simulink model "Deadbeat_controller"  (R2021b)
settings: Solver=ode45  StartTime=0.0  StopTime=0.5  RelTol=1e-3
values from neighbouring files (symbols this model uses):
  G1 = 1/(R + L*s)    [Project.m]
  G2 = Kt/(m*s^2 + c*s + k)    [Project.m]
  Gd_db = minreal(Fz/(Gz * (1 - Fz)))    [Project.m]
  Ts = 0.02    [Project.m]
settings Model: Creator=Amir  LastModifiedBy=Amir

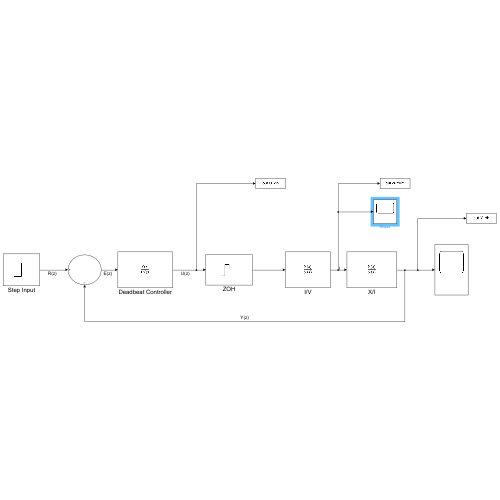
[thumbnail: Simulink's stored preview of the top-level diagram]
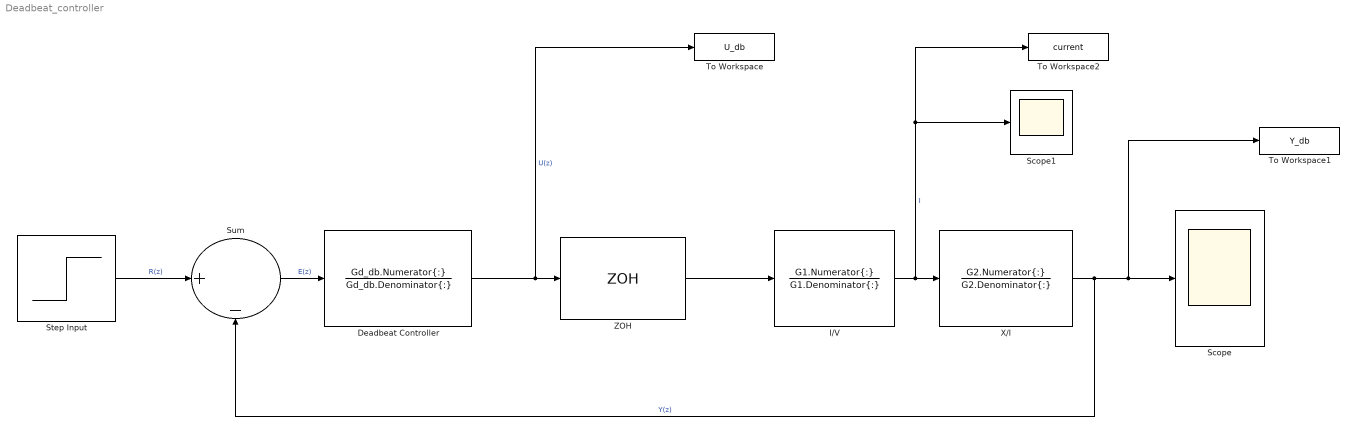
== system Deadbeat_controller ==
  Deadbeat Controller : DiscreteTransferFcn  Numerator=Gd_db.Numerator{:}  Denominator=Gd_db.Denominator{:}  SampleTime=Ts
  I/V : TransferFcn  Numerator=G1.Numerator{:}  Denominator=G1.Denominator{:}
  Scope : Scope
  Scope1 : Scope
  Step Input : Step  Time=0  After=0.01  SampleTime=0
  Sum : Sum  Inputs=|+-
  To Workspace : ToWorkspace  VariableName=U_db  SaveFormat=Timeseries  SampleTime=-1
  To Workspace1 : ToWorkspace  VariableName=Y_db  SaveFormat=Timeseries  SampleTime=-1
  To Workspace2 : ToWorkspace  VariableName=current  SaveFormat=Timeseries  SampleTime=-1
  X/I : TransferFcn  Numerator=G2.Numerator{:}  Denominator=G2.Denominator{:}
  ZOH : ZeroOrderHold  SampleTime=Ts
  wires:
  Deadbeat Controller/1 -> To Workspace/1, ZOH/1  "U(z)"
  ZOH/1 -> I/V/1
  X/I/1 -> Sum/2, To Workspace1/1, Scope/1  "Y(z)"
  Step Input/1 -> Sum/1  "R(z)"
  Sum/1 -> Deadbeat Controller/1  "E(z)"
  I/V/1 -> Scope1/1, To Workspace2/1, X/I/1  "I"
